simulink subsystem "testSelector"  (R2023a)
settings: Solver=VariableStepAuto  StartTime=0.0  StopTime=10.0  RelTol=1e-3
model mask{amp1=12, amp2=12, amp3=12}
  mask prompts: amp1 "Коэффициент усиления"; amp2 "Амплитуда синусоидального входного сигнала"; amp3 "Амплитуда импульсного воздействия"
settings Model: Creator=diontep  LastModifiedBy=diontep

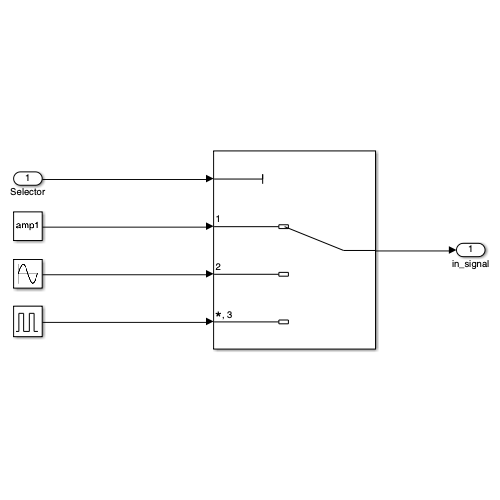
[thumbnail: Simulink's stored preview of the top-level diagram]
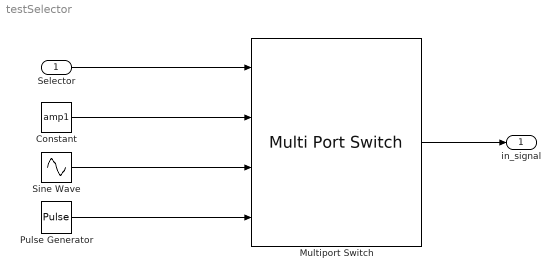
== system testSelector ==
  Selector : Inport
  Constant : Constant  Value=amp1
  Multiport Switch : MultiPortSwitch  SaturateOnIntegerOverflow=off  InputSameDT=off
  Pulse Generator : DiscretePulseGenerator  PulseType=Time based  Amplitude=amp3  Period=0.5  PulseWidth=5
  Sine Wave : Sin  Amplitude=amp2  Frequency=0.5  SampleTime=0
  in_signal : Outport
  wires:
  Pulse Generator/1 -> Multiport Switch/4
  Selector/1 -> Multiport Switch/1
  Constant/1 -> Multiport Switch/2
  Sine Wave/1 -> Multiport Switch/3
  Multiport Switch/1 -> in_signal/1
